simulink model "test_spring_stiffness"  (R2014b)
settings: Solver=FixedStepDiscrete  StartTime=0.0  StopTime=inf  FixedStep=sample_time  RelTol=1e-3
StartFcn:
  | tg.sampletime = correctedSampleTime;
settings Model: SimulationMode=external  BufferReuse=off  Creator=wmartin  LastModifiedBy=drl
settings SolverCC: EnableConcurrentExecution=on
settings DataIOCC: LimitDataPoints=off  MaxDataPoints=1e7  SaveFormat=StructureWithTime  SignalLogging=off  DSMLogging=off
settings OptimizationCC: BlockReduction=off  OptimizeBlockIOStorage=off  BufferReuse=off  GlobalBufferReuse=off  ExpressionFolding=off  ExpressionDepthLimit=2147483647  LocalBlockOutputs=off  SimCompilerOptimization=On  AccelVerboseBuild=on
settings DebuggingCC: UnderspecifiedInitializationDetection=Classic  MergeDetectMultiDrivingBlocksExec=none  StateNameClashWarn=warning
settings HardwareCC: ProdIntDivRoundTo=Zero  ProdEndianess=LittleEndian  ProdLongLongMode=on  ProdHWDeviceType=Generic->32-bit x86 compatible
settings ModelReferenceCC: UpdateModelReferenceTargets=IfOutOfDate  EnableParallelModelReferenceBuilds=on  ModelReferenceNumInstancesAllowed=Single  ModelReferenceMinAlgLoopOccurrences=on
settings RTWCC: SystemTargetFile=slrt.tlc  TemplateMakefile=slrt_default_tmf  Description=Simulink Real-Time  RTWVerbose=off  ProcessScript=slrt_make_rtw_hook  CodeProfilingSaveOptions=AllData  RTWCompilerOptimization=On
settings CodeAppCC: GenerateComments=off  MaxIdLength=256  SimulinkBlockComments=off
settings SimulinkRealTimeCC: GeneratePreprocessorConditionals=Disable all  EnableShiftOperators=on  RL32LogBufSizeModifier=1e8

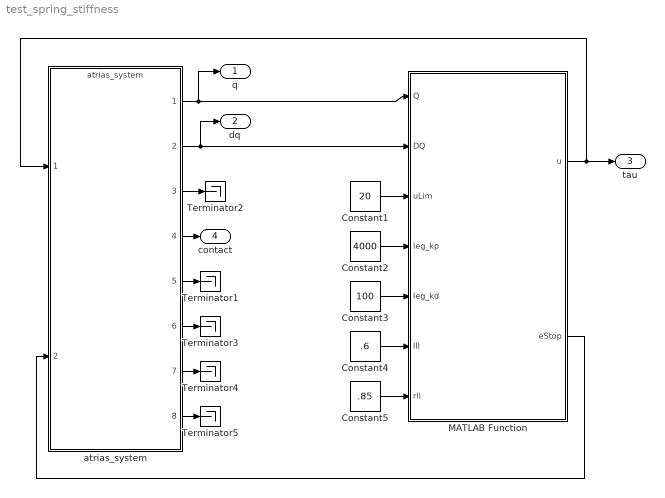
== system test_spring_stiffness ==
  Constant1 : Constant  Value=20
  Constant2 : Constant  Value=4000
  Constant3 : Constant  Value=100
  Constant4 : Constant  Value=.6
  Constant5 : Constant  Value=.85
  MATLAB Function : MATLAB Function  TreatAsAtomicUnit=on
  Terminator{1..5} (5 alike) : Terminator
  atrias_system : ModelReference  ModelNameDialog=atrias_system  SimulationMode=Normal  ModelReferenceVersion=1.2413  CopyOfModelName=atrias_system  DefaultDataLogging=on
  q : Outport
  dq : Outport  Port=2
  tau : Outport  Port=3
  contact : Outport  Port=4
  wires:
  atrias_system/2 -> dq/1, MATLAB Function/2(DQ)
  MATLAB Function/1(u) -> atrias_system/1, tau/1
  MATLAB Function/2(eStop) -> atrias_system/2
  atrias_system/3 -> Terminator2/1
  atrias_system/1 -> q/1, MATLAB Function/1(Q)
  Constant1/1 -> MATLAB Function/3(uLim)
  Constant2/1 -> MATLAB Function/4(leg_kp)
  Constant3/1 -> MATLAB Function/5(leg_kd)
  Constant4/1 -> MATLAB Function/6(lll)
  Constant5/1 -> MATLAB Function/7(rll)
  atrias_system/4 -> contact/1
  atrias_system/5 -> Terminator1/1
  atrias_system/6 -> Terminator3/1
  atrias_system/7 -> Terminator4/1
  atrias_system/8 -> Terminator5/1

== matlab function test_spring_stiffness/MATLAB Function ==
  data: Q input; u output; DQ input; eStop output; uLim input; leg_kp input; leg_kd input; lll input; rll input
function [u, eStop] = springTestController(Q, DQ, uLim, leg_kp, leg_kd, lll, rll)
%SPRINGTESTCONTROLLER Spring stiffness testing controller.
%
% Description:
%
% Notes:
% 	- State indexes (rBl rBm rAl rAm lBl lBm lAl lAm rHm lHm bR bY bP) 
%   - Input indexes (rB rA rH lB lA lH)

    % Set default emergency stop to false
    eStop = false;
    
    % Define actuator gains
    hip_kp = 1500; hip_kd = 50;
    
    % Initialize input vector to zeros
    u = zeros(6,1);
  
    % Check inputs
    lll = clamp(lll, 0.5, 0.95);
    rll = clamp(rll, 0.5, 0.95);
    
	% Compute hip actuator torques using PD controller
	u([3 6]) = (0 - Q([9 10]))*hip_kp + (0 - DQ([9 10]))*hip_kd;
    
    % Compute leg actuator torques using PD controller
    x0 = pi + [acos(rll); -acos(rll); acos(lll); -acos(lll)];
    u([1 2 4 5]) = (x0 - Q([2 4 6 8]))*leg_kp + (0 - DQ([2 4 6 8]))*leg_kd;

    % Limit torques to be cautious
	u = clamp(u, -uLim, uLim);
end % springTestController

function b = clamp(a, lim1, lim2)
%CLAMP Clamp value between two values.
	
	% Find which limit is min and max
	aMin = min([lim1, lim2]);
	aMax = max([lim1, lim2]);

	% Clamp value between limits
	b = max(min(a, aMax), aMin);
end % clamp
